simulink model "MPC_CONTROLLED"  (R2023b)
settings: Solver=FixedStepAuto  StartTime=0.0  StopTime=10  FixedStep=0.002  RelTol=1e-3
settings Model: Creator=franc  LastModifiedBy=franc

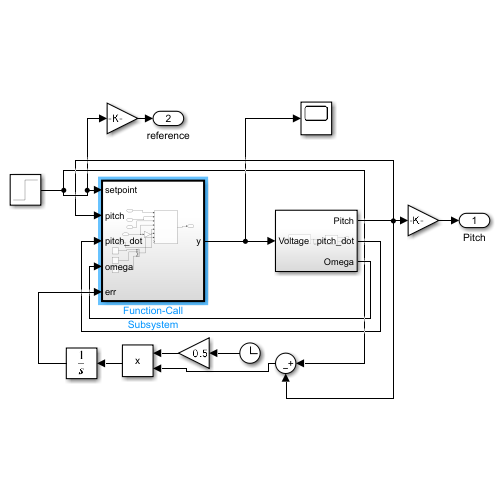
[thumbnail: Simulink's stored preview of the top-level diagram]
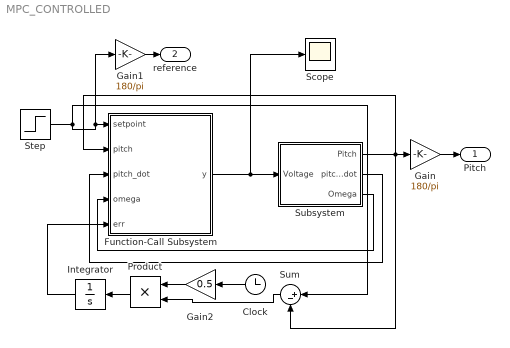
== system MPC_CONTROLLED ==
  Clock : Clock
  Function-Call Subsystem : Subsystem  TreatAsAtomicUnit=on  SystemSampleTime=0.1
  Gain : Gain  Gain=180/pi
  Gain1 : Gain  Gain=180/pi
  Gain2 : Gain  Gain=0.5
  Integrator : Integrator
  Product : Product
  Scope : Scope
  Step : Step  After=pi/6  SampleTime=0
  Subsystem : Subsystem
  Sum : Sum  Inputs=|+-
  Pitch : Outport
  reference : Outport  Port=2
  wires:
  Subsystem/2(pitch_dot) -> Function-Call Subsystem/3(pitch_dot)
  Subsystem/3(Omega) -> Function-Call Subsystem/4(omega)
  Step/1 -> Gain1/1, Function-Call Subsystem/1(setpoint), Sum/1
  Subsystem/1(Pitch) -> Sum/2, Gain/1, Function-Call Subsystem/2(pitch)
  Function-Call Subsystem/1(y) -> Scope/1, Subsystem/1(Voltage)
  Gain/1 -> Pitch/1
  Gain1/1 -> reference/1
  Integrator/1 -> Function-Call Subsystem/5(err)
  Sum/1 -> Product/2
  Product/1 -> Integrator/1
  Clock/1 -> Gain2/1
  Gain2/1 -> Product/1

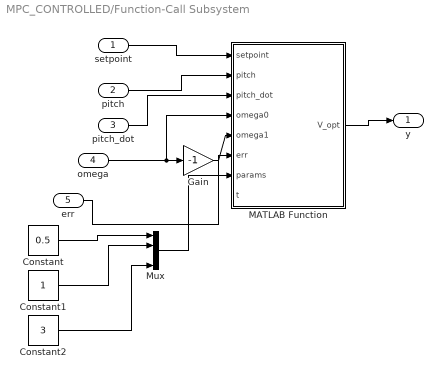
== system MPC_CONTROLLED/Function-Call Subsystem ==
  setpoint : Inport
  pitch : Inport  Port=2
  pitch_dot : Inport  Port=3
  omega : Inport  Port=4
  err : Inport  Port=5
  Constant : Constant  Value=0.5
  Constant1 : Constant
  Constant2 : Constant  Value=3
  Gain : Gain  Gain=-1
  MATLAB Function : MATLAB Function  TreatAsAtomicUnit=on
  Mux : Mux
  y : Outport
  wires:
  setpoint/1 -> MATLAB Function/1(setpoint)
  pitch/1 -> MATLAB Function/2(pitch)
  pitch_dot/1 -> MATLAB Function/3(pitch_dot)
  omega/1 -> Gain/1, MATLAB Function/4(omega0)
  MATLAB Function/1(V_opt) -> y/1
  err/1 -> MATLAB Function/6(err)
  Gain/1 -> MATLAB Function/5(omega1)
  Constant/1 -> Mux/1
  Mux/1 -> MATLAB Function/7(params)
  Constant1/1 -> Mux/2
  Constant2/1 -> Mux/4

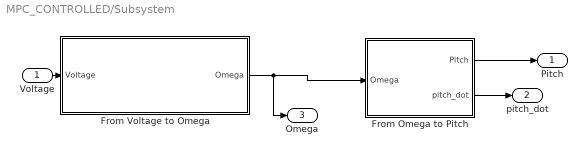
== system MPC_CONTROLLED/Subsystem ==
  Voltage : Inport
  From Omega to Pitch : Subsystem
  From Voltage to Omega : Subsystem
  Pitch : Outport
  pitch_dot : Outport  Port=2
  Omega : Outport  Port=3
  wires:
  From Voltage to Omega/1(Omega) -> Omega/1, From Omega to Pitch/1(Omega)
  Voltage/1 -> From Voltage to Omega/1(Voltage)
  From Omega to Pitch/1(Pitch) -> Pitch/1
  From Omega to Pitch/2(pitch_dot) -> pitch_dot/1

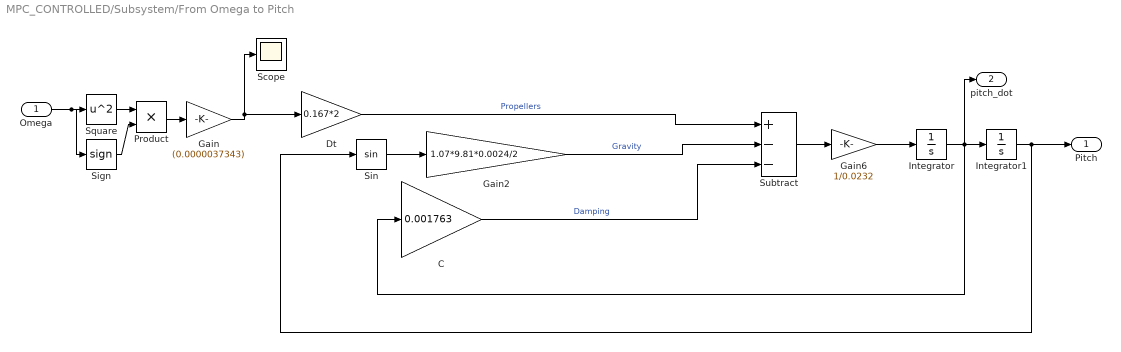
== system MPC_CONTROLLED/Subsystem/From Omega to Pitch ==
  Omega : Inport
  C : Gain  Gain=0.001763
  Dt : Gain  Gain=0.167*2
  Gain : Gain  Gain=(0.0000037343)
  Gain2 : Gain  Gain=1.07*9.81*0.0024/2
  Gain6 : Gain  Gain=1/0.0232
  Integrator : Integrator
  Integrator1 : Integrator
  Product : Product
  Scope : Scope
  Sign : Signum  ZeroCross=off
  Sin : Trigonometry
  Square : Math  Operator=square
  Subtract : Sum  Inputs=+--
  Pitch : Outport
  pitch_dot : Outport  Port=2
  wires:
  Integrator1/1 -> Pitch/1, Sin/1
  Sin/1 -> Gain2/1
  Subtract/1 -> Gain6/1
  Gain2/1 -> Subtract/2  "Gravity"
  C/1 -> Subtract/3  "Damping"
  Omega/1 -> Sign/1, Square/1
  Gain6/1 -> Integrator/1
  Integrator/1 -> pitch_dot/1, Integrator1/1, C/1
  Dt/1 -> Subtract/1  "Propellers"
  Product/1 -> Gain/1
  Square/1 -> Product/1
  Sign/1 -> Product/2
  Gain/1 -> Scope/1, Dt/1

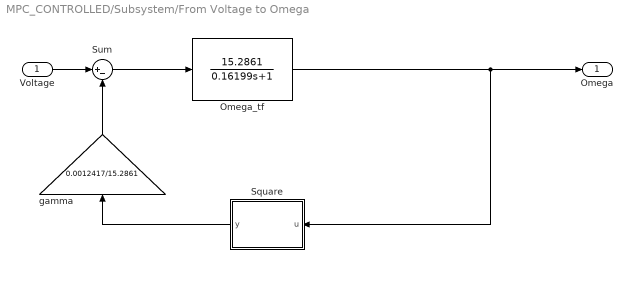
== system MPC_CONTROLLED/Subsystem/From Voltage to Omega ==
  Voltage : Inport
  Omega_tf : TransferFcn  Numerator=15.2861  Denominator=[0.16199 1]
  Square : MATLAB Function  TreatAsAtomicUnit=on
  Sum : Sum  Inputs=|+-
  gamma : Gain  Gain=0.0012417/15.2861
  Omega : Outport
  wires:
  Voltage/1 -> Sum/1
  gamma/1 -> Sum/2
  Square/1(y) -> gamma/1
  Omega_tf/1 -> Omega/1, Square/1(u)
  Sum/1 -> Omega_tf/1

== matlab function MPC_CONTROLLED/Function-Call Subsystem/MATLAB Function ==
  data: setpoint input; V_opt output; pitch input; pitch_dot input; omega0 input; omega1 input; err input; params input; t input
function V_opt  = asyncFunction(setpoint,pitch,pitch_dot,omega0,omega1, err,params,t)
    fun=@(V)simulate_pitch(0.1,[omega0,omega1,pitch_dot,pitch,err],V,setpoint,0,params,t);
    opts=optimoptions("fmincon","Algorithm","sqp","MaxFunctionEvaluations",1e5);
    size=10;
    V_opt_full=fmincon(fun,1*ones(size,1),[eye(size);-eye(size)],[18*ones(size,1);18*ones(size,1)],[],[],[],[],[],opts);
    V_opt=mean(V_opt_full(1));
end

== matlab function MPC_CONTROLLED/Subsystem/From Voltage to Omega/Square ==
  data: u input; y output
function y = fcn(u)
y=u^2*sign(u);
